simulink model "InputOutput_linearization"  (R2024b)
settings: Solver=VariableStepAuto  StartTime=0.0  StopTime=T  FixedStep=Ts  RelTol=1e-3
InitFcn:
  | cubic_polynomial;
StopFcn:
  | plotting;
values from neighbouring files (symbols this model uses):
  b = 0.1    [cubic_polynomial.m]
  k1 = 2    [cubic_polynomial.m]
  k2 = 2    [cubic_polynomial.m]
  Ts = 0.01    [cubic_polynomial.m]
libraries: robotmobilelib x1
settings Model: Creator=salva  LastModifiedBy=salva

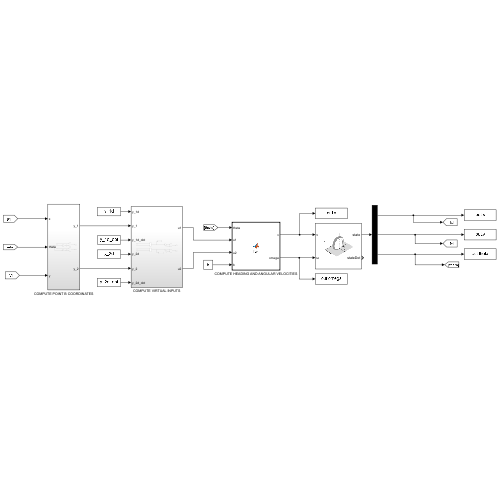
[thumbnail: Simulink's stored preview of the top-level diagram]
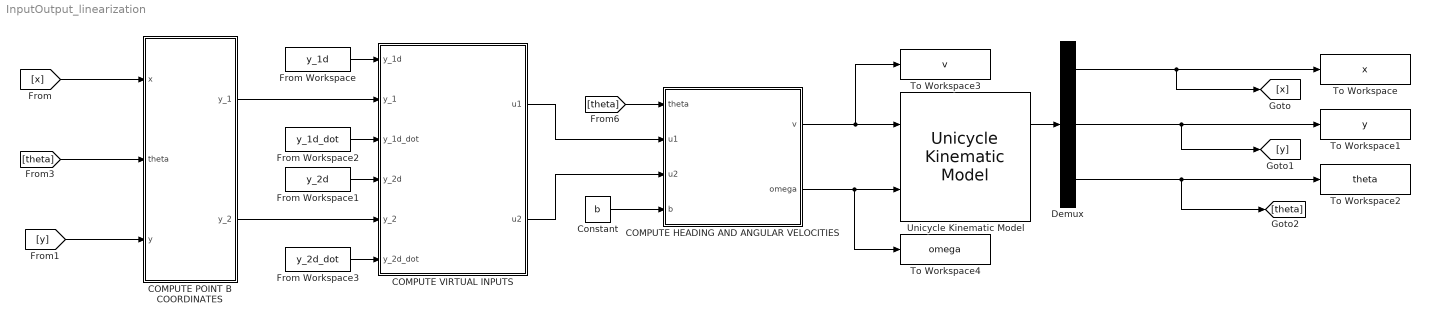
== system InputOutput_linearization ==
  COMPUTE HEADING AND ANGULAR VELOCITIES : MATLAB Function  TreatAsAtomicUnit=on
  COMPUTE POINT B COORDINATES : Subsystem
  COMPUTE VIRTUAL INPUTS : Subsystem
  Constant : Constant  Value=b
  Demux : Demux  Outputs=3
  From Workspace : FromWorkspace  VariableName=y_1d
  From Workspace1 : FromWorkspace  VariableName=y_2d
  From Workspace2 : FromWorkspace  VariableName=y_1d_dot
  From Workspace3 : FromWorkspace  VariableName=y_2d_dot
  To Workspace : ToWorkspace  VariableName=x  SaveFormat=Timeseries  SampleTime=Ts
  To Workspace1 : ToWorkspace  VariableName=y  SaveFormat=Timeseries  SampleTime=Ts
  To Workspace2 : ToWorkspace  VariableName=theta  SaveFormat=Timeseries  SampleTime=Ts
  To Workspace3 : ToWorkspace  VariableName=v  SaveFormat=Timeseries  SampleTime=Ts
  To Workspace4 : ToWorkspace  VariableName=omega  SaveFormat=Timeseries  SampleTime=Ts
  Unicycle Kinematic Model : robotmobilelib/Unicycle Kinematic Model  VehicleInputs=Vehicle Speed & Heading Angular Velocity  WheelRadius=0.25  WheelSpeedRange=[-Inf Inf]  InitialState=[0; 0; 0]  SimulateUsing=Interpreted execution
  wires:
  Unicycle Kinematic Model/1 -> Demux/1
  Demux/1 -> [x], To Workspace/1
  Demux/2 -> [y], To Workspace1/1
  Demux/3 -> To Workspace2/1, [theta]
  From Workspace/1 -> COMPUTE VIRTUAL INPUTS/1(y_1d)
  COMPUTE POINT B COORDINATES/1(y_1) -> COMPUTE VIRTUAL INPUTS/2(y_1)
  From Workspace2/1 -> COMPUTE VIRTUAL INPUTS/3(y_1d_dot)
  From Workspace1/1 -> COMPUTE VIRTUAL INPUTS/4(y_2d)
  From Workspace3/1 -> COMPUTE VIRTUAL INPUTS/6(y_2d_dot)
  [x] -> COMPUTE POINT B COORDINATES/1(x)
  [theta] -> COMPUTE POINT B COORDINATES/2(theta)
  [y] -> COMPUTE POINT B COORDINATES/3(y)
  COMPUTE POINT B COORDINATES/2(y_2) -> COMPUTE VIRTUAL INPUTS/5(y_2)
  COMPUTE HEADING AND ANGULAR VELOCITIES/1(v) -> To Workspace3/1, Unicycle Kinematic Model/1
  COMPUTE HEADING AND ANGULAR VELOCITIES/2(omega) -> To Workspace4/1, Unicycle Kinematic Model/2
  [theta] -> COMPUTE HEADING AND ANGULAR VELOCITIES/1(theta)
  COMPUTE VIRTUAL INPUTS/1(u1) -> COMPUTE HEADING AND ANGULAR VELOCITIES/2(u1)
  COMPUTE VIRTUAL INPUTS/2(u2) -> COMPUTE HEADING AND ANGULAR VELOCITIES/3(u2)
  Constant/1 -> COMPUTE HEADING AND ANGULAR VELOCITIES/4(b)

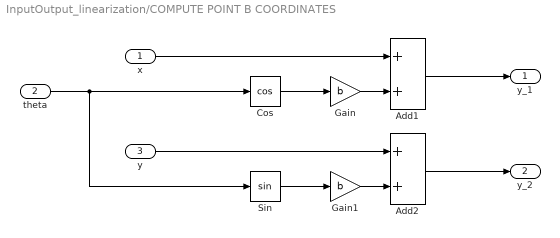
== system InputOutput_linearization/COMPUTE POINT B COORDINATES ==
  x : Inport
  theta : Inport  Port=2
  y : Inport  Port=3
  Add1 : Sum
  Add2 : Sum
  Cos : Trigonometry  Operator=cos
  Gain : Gain  Gain=b
  Gain1 : Gain  Gain=b
  Sin : Trigonometry
  y_1 : Outport
  y_2 : Outport  Port=2
  wires:
  Sin/1 -> Gain1/1
  Gain/1 -> Add1/2
  Gain1/1 -> Add2/2
  y/1 -> Add2/1
  x/1 -> Add1/1
  Cos/1 -> Gain/1
  theta/1 -> Cos/1, Sin/1
  Add1/1 -> y_1/1
  Add2/1 -> y_2/1

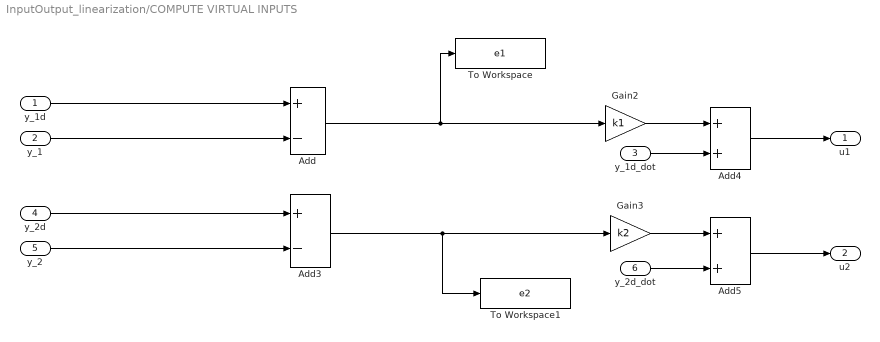
== system InputOutput_linearization/COMPUTE VIRTUAL INPUTS ==
  y_1d : Inport
  y_1 : Inport  Port=2
  y_1d_dot : Inport  Port=3
  y_2d : Inport  Port=4
  y_2 : Inport  Port=5
  y_2d_dot : Inport  Port=6
  Add : Sum  Inputs=+-
  Add3 : Sum  Inputs=+-
  Add4 : Sum
  Add5 : Sum
  Gain2 : Gain  Gain=k1
  Gain3 : Gain  Gain=k2
  To Workspace : ToWorkspace  VariableName=e1  SaveFormat=Timeseries  SampleTime=Ts
  To Workspace1 : ToWorkspace  VariableName=e2  SaveFormat=Timeseries  SampleTime=Ts
  u1 : Outport
  u2 : Outport  Port=2
  wires:
  Gain2/1 -> Add4/1
  Gain3/1 -> Add5/1
  y_2/1 -> Add3/2
  Add3/1 -> To Workspace1/1, Gain3/1
  Add/1 -> To Workspace/1, Gain2/1
  Add5/1 -> u2/1
  Add4/1 -> u1/1
  y_1d_dot/1 -> Add4/2
  y_1d/1 -> Add/1
  y_2d/1 -> Add3/1
  y_2d_dot/1 -> Add5/2
  y_1/1 -> Add/2

== matlab function InputOutput_linearization/COMPUTE HEADING AND ANGULAR VELOCITIES ==
  data: theta input; v output; u1 input; u2 input; b input; omega output
function [v,omega]  = fcn(theta,u1,u2,b)

    T_theta_inv=inv([cos(theta),-b*sin(theta);
        sin(theta),b*cos(theta)]);

    res=T_theta_inv*[u1;u2];

    v=res(1);
    omega=res(2);
    
end
